simulink model "flexibleMissile"  (R2015a)
settings: Solver=ode45  StartTime=0.0  StopTime=10.0  RelTol=1e-3
values from neighbouring files (symbols this model uses):
  flexi = flexi({'\varepsilon_{46}';'q_{10}';'q_{83}';'a_{z10}';'a_{z53}';'a_{z83}';'a_{z92}'},'F_{1}')    [initFlexibleModel.m]
  T0 = double(T0)    [getRigidBodySS.m]
settings Model: CovSFcnEnable=off  Creator=s220385  LastModifiedBy=anatole
settings DebuggingCC: SolverPrmCheckMsg=warning

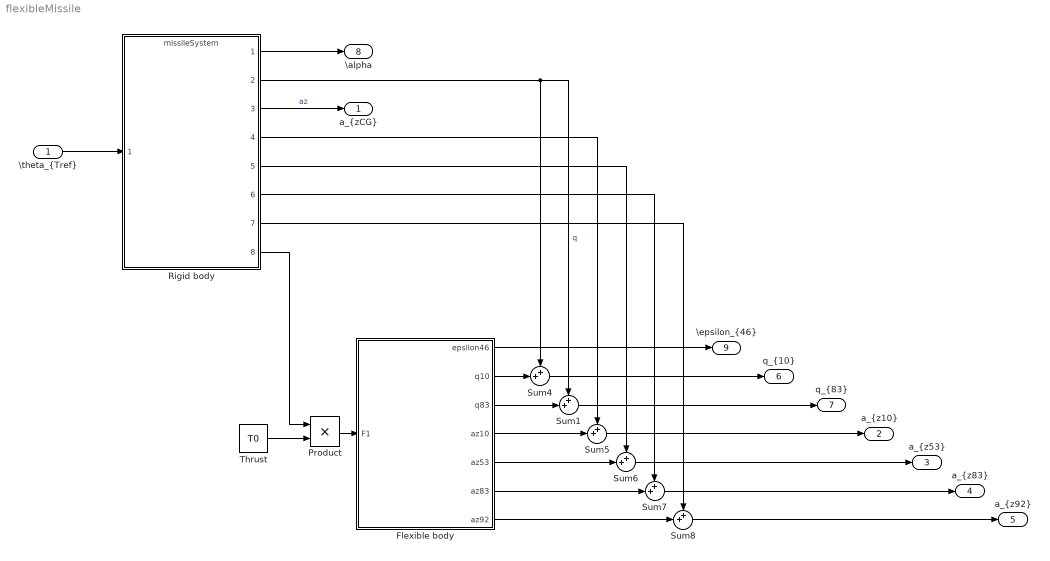
== system flexibleMissile ==
  "\\theta_{Tref}" : Inport
  Flexible body : Subsystem
      mask Display:
      | port_label('input',1,'Lateral Thrust')
      | 
      | port_label('output',1,'\epsilon_{46}','texmode','on')
      | port_label('output',2,'q_{10}','texmode','on')
      | port_label('output',3,'q_{83}','texmode','on')
      | port_label('output',4,'a_{z10}','texmode','on')
      | port_label('output',5,'a_{z53}','texmode','on')
      | port_label('output',6,'a_{z83}','texmode','on')
      | port_label('output',7,'a_{z92}','texmode','on')
  Product : Product
  Rigid body : ModelReference  ModelNameDialog=missileSystem  SimulationMode=Normal  ModelReferenceVersion=1.13  CopyOfModelName=missileSystem  DefaultDataLogging=on
      mask Display:
      | port_label('input',1,'\theta_{Tref}','texmode','on')
      | 
      | port_label('output',1,'\alpha','texmode','on')
      | port_label('output',2,'q','texmode','on')
      | port_label('output', 3, 'a_{zCG}','texmode','on')
      | port_label('output', 4, 'a_{z10}','texmode','on')
      | port_label('output', 5, 'a_{z53}','texmode','on')
      | port_label('output', 6, 'a_{z83}','texmode','on')
      | port_label('output', 7, 'a_{z91}','texmode','on')
      | port_label('output',8,'\theta_T','texmode','on')
  Sum{1,4..8} (6 alike) : Sum  Inputs=++|
  Thrust : Constant  Value=T0
  "a_{zCG}" : Outport
  "a_{z10}" : Outport  Port=2
  "a_{z53}" : Outport  Port=3
  "a_{z83}" : Outport  Port=4
  "a_{z92}" : Outport  Port=5
  "q_{10}" : Outport  Port=6
  "q_{83}" : Outport  Port=7
  \alpha : Outport  Port=8
  "\\epsilon_{46}" : Outport  Port=9
  wires:
  Product/1 -> Flexible body/1(F1)
  Thrust/1 -> Product/2
  "\\theta_{Tref}"/1 -> Rigid body/1
  Rigid body/1 -> \alpha/1
  Rigid body/8 -> Product/1
  Flexible body/3(q83) -> Sum1/2
  Flexible body/4(az10) -> Sum5/2
  Flexible body/5(az53) -> Sum6/2
  Flexible body/6(az83) -> Sum7/2
  Flexible body/7(az92) -> Sum8/2
  Flexible body/2(q10) -> Sum4/2
  Rigid body/2 -> Sum1/1, Sum4/1  "q"
  Rigid body/4 -> Sum5/1
  Rigid body/5 -> Sum6/1
  Rigid body/6 -> Sum7/1
  Rigid body/7 -> Sum8/1
  Rigid body/3 -> "a_{zCG}"/1  "az"
  Flexible body/1(epsilon46) -> "\\epsilon_{46}"/1
  Sum4/1 -> "q_{10}"/1
  Sum1/1 -> "q_{83}"/1
  Sum5/1 -> "a_{z10}"/1
  Sum6/1 -> "a_{z53}"/1
  Sum7/1 -> "a_{z83}"/1
  Sum8/1 -> "a_{z92}"/1

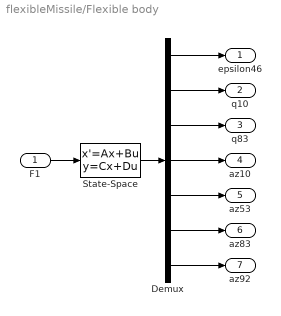
== system flexibleMissile/Flexible body ==
  F1 : Inport
  Demux : Demux  Outputs=7
  State-Space : StateSpace  A=flexi.a  B=flexi.b  C=flexi.c  D=flexi.d  X0=0
  epsilon46 : Outport
  q10 : Outport  Port=2
  q83 : Outport  Port=3
  az10 : Outport  Port=4
  az53 : Outport  Port=5
  az83 : Outport  Port=6
  az92 : Outport  Port=7
  wires:
  F1/1 -> State-Space/1
  State-Space/1 -> Demux/1
  Demux/1 -> epsilon46/1
  Demux/2 -> q10/1
  Demux/3 -> q83/1
  Demux/4 -> az10/1
  Demux/5 -> az53/1
  Demux/6 -> az83/1
  Demux/7 -> az92/1
